simulink model "Simulation5"  (R2020a)
settings: Solver=VariableStepAuto  StartTime=0.0  StopTime=1*60*24  RelTol=1e-3
model workspace (MAT data in the model file):
  hr = 0
  mn = 0
libraries: fl_lib x75, nesl_utility x45, simulink_extras x8
(part 2 of 2)

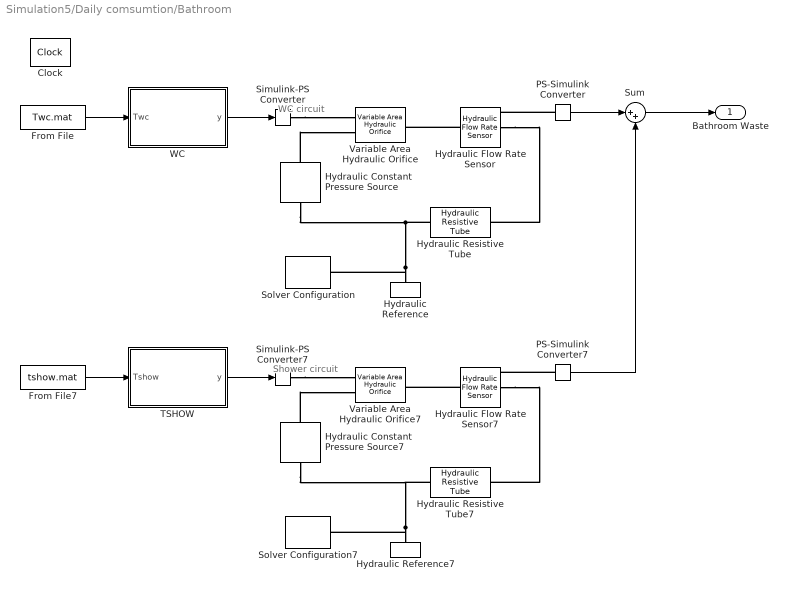
== system Simulation5/Daily comsumtion/Bathroom ==
  note: WC circuit
  note: Shower circuit
  Clock : simulink_extras/Flip Flops/Clock  period=1
  From File : FromFile  FileName=Twc.mat  SampleTime=0
  From File7 : FromFile  FileName=tshow.mat  SampleTime=0
  Hydraulic Constant Pressure Source : fl_lib/Hydraulic/Hydraulic Sources/Hydraulic Constant Pressure Source  commanded_pressure=3 bar
      settings: SourceProductBaseCode=SS  InternalSimscapePortConfiguration="{\"Bottom\":[],\"Left\":[{\"id\":\"P\",\"label\":\"P\",\"type\":\"foundation.hydraulic.hydraulic\"}],\"Right\":[{\"id\":\"T\",\"label\":\"T\",\"type\":\"foundation.hydraulic.hydraulic\"}],\"Top\":[]}"
  Hydraulic Constant Pressure Source7 : fl_lib/Hydraulic/Hydraulic Sources/Hydraulic Constant Pressure Source  commanded_pressure=3 bar
      settings: SourceProductBaseCode=SS  InternalSimscapePortConfiguration="{\"Bottom\":[],\"Left\":[{\"id\":\"P\",\"label\":\"P\",\"type\":\"foundation.hydraulic.hydraulic\"}],\"Right\":[{\"id\":\"T\",\"label\":\"T\",\"type\":\"foundation.hydraulic.hydraulic\"}],\"Top\":[]}"
  Hydraulic Flow Rate Sensor : fl_lib/Hydraulic/Hydraulic Sensors/Hydraulic Flow Rate Sensor
  Hydraulic Flow Rate Sensor7 : fl_lib/Hydraulic/Hydraulic Sensors/Hydraulic Flow Rate Sensor
  Hydraulic Reference : fl_lib/Hydraulic/Hydraulic Elements/Hydraulic Reference
  Hydraulic Reference7 : fl_lib/Hydraulic/Hydraulic Elements/Hydraulic Reference
  Hydraulic Resistive Tube : fl_lib/Hydraulic/Hydraulic Elements/Hydraulic Resistive Tube  cs_type=1  d_in=19 mm  area=1e-4 m^2  D_h=1.12e-2 m  s_factor=0.032  length=17 m  length_ad=1 m  roughness=15e-6 m  Re_lam=2000  Re_turb=4000  q_specify=off  q_priority=None  q=0.001 m^3/s  q_nominal_specify=off  q_nominal_unit=m^3/s  q_nominal_value=1  p_specify=off  p_priority=None  p=0 Pa  p_nominal_specify=off  p_nominal_unit=Pa  p_nominal_value=1
      settings: SourceProductBaseCode=SS  InternalSimscapePortConfiguration="{\"Bottom\":[],\"Left\":[{\"id\":\"A\",\"label\":\"A\",\"type\":\"foundation.hydraulic.hydraulic\"}],\"Right\":[{\"id\":\"B\",\"label\":\"B\",\"type\":\"foundation.hydraulic.hydraulic\"}],\"Top\":[]}"
  Hydraulic Resistive Tube7 : fl_lib/Hydraulic/Hydraulic Elements/Hydraulic Resistive Tube  cs_type=1  d_in=19 mm  area=1e-4 m^2  D_h=1.12e-2 m  s_factor=64  length=17 m  length_ad=1 m  roughness=15e-6 m  Re_lam=2000  Re_turb=4000  q_specify=off  q_priority=None  q=0.001 m^3/s  q_nominal_specify=off  q_nominal_unit=m^3/s  q_nominal_value=1  p_specify=off  p_priority=None  p=0 Pa  p_nominal_specify=off  p_nominal_unit=Pa  p_nominal_value=1
      settings: SourceProductBaseCode=SS  InternalSimscapePortConfiguration="{\"Bottom\":[],\"Left\":[{\"id\":\"A\",\"label\":\"A\",\"type\":\"foundation.hydraulic.hydraulic\"}],\"Right\":[{\"id\":\"B\",\"label\":\"B\",\"type\":\"foundation.hydraulic.hydraulic\"}],\"Top\":[]}"
  PS-Simulink Converter : nesl_utility/PS-Simulink Converter  PhysicalDomain=network_engine_domain  SubClassName=ps_output  LeftPortType=input  RightPortType=output  PseudoPeriodic=off  Frequencies=[]  Unit=1  AffineConversion=off
  PS-Simulink Converter7 : nesl_utility/PS-Simulink Converter  PhysicalDomain=network_engine_domain  SubClassName=ps_output  LeftPortType=input  RightPortType=output  PseudoPeriodic=off  Frequencies=[]  Unit=1  AffineConversion=off
  Simulink-PS Converter : nesl_utility/Simulink-PS Converter  PhysicalDomain=network_engine_domain  SubClassName=ps_input  LeftPortType=input  RightPortType=output  PseudoPeriodic=off  Frequencies=[]  NoiseDistribution=none  NoiseParameters=[]  Unit=1  AffineConversion=off  FilteringAndDerivatives=provide  SimscapeFilterOrder=1  InputFilterTimeConstant=0.001  UdotUserProvided=0
  Simulink-PS Converter7 : nesl_utility/Simulink-PS Converter  PhysicalDomain=network_engine_domain  SubClassName=ps_input  LeftPortType=input  RightPortType=output  PseudoPeriodic=off  Frequencies=[]  NoiseDistribution=none  NoiseParameters=[]  Unit=1  AffineConversion=off  FilteringAndDerivatives=provide  SimscapeFilterOrder=1  InputFilterTimeConstant=0.001  UdotUserProvided=0
  Solver Configuration : nesl_utility/Solver Configuration  PhysicalDomain=network_engine_domain  SubClassName=solver  LeftPortType=input  RightPortType=generic  Tones=[]  Harmonics=[]  SimulateNoise=off  Profile=off  UseLocalSampling=off  EnableSwitchedLinearOptims=on  FrequencyDomain=off  UseCCode=off  RelTol=0.001  AbsTol=1e-06  MinStep=1e-09  ToWorkspace=off  RevertToSquareIcSolve=off  NumHomotopyIterations=100  PhasorMode=off  PhasorModeNumHarmonics=1  DoDC=off  ResidualTolerance=1e-09  UseLocalSolver=off  LocalSolverChoice=NE_BACKWARD_EULER_ADVANCER  LocalSolverSampleTime=0.001  DoFixedCost=off  MaxNonlinIter=3  MaxModeIter=2  LinearAlgebra=auto  EquationFormulation=NE_TIME_EF  DelaysMemoryBudget=1024  AutomaticFiltering=on  FilteringTimeConstant=0.001  PartitionStorageMethod=AS_NEEDED  PartitionMemoryBudget=1024  PartitionMethod=ROBUST
  Solver Configuration7 : nesl_utility/Solver Configuration  PhysicalDomain=network_engine_domain  SubClassName=solver  LeftPortType=input  RightPortType=generic  Tones=[]  Harmonics=[]  SimulateNoise=off  Profile=off  UseLocalSampling=off  EnableSwitchedLinearOptims=on  FrequencyDomain=off  UseCCode=off  RelTol=0.001  AbsTol=1e-06  MinStep=1e-09  ToWorkspace=off  RevertToSquareIcSolve=off  NumHomotopyIterations=100  PhasorMode=off  PhasorModeNumHarmonics=1  DoDC=off  ResidualTolerance=1e-09  UseLocalSolver=off  LocalSolverChoice=NE_BACKWARD_EULER_ADVANCER  LocalSolverSampleTime=0.001  DoFixedCost=off  MaxNonlinIter=3  MaxModeIter=2  LinearAlgebra=auto  EquationFormulation=NE_TIME_EF  DelaysMemoryBudget=1024  AutomaticFiltering=on  FilteringTimeConstant=0.001  PartitionStorageMethod=AS_NEEDED  PartitionMemoryBudget=1024  PartitionMethod=ROBUST
  Sum : Sum  Inputs=|++
  TSHOW : MATLAB Function  TreatAsAtomicUnit=on
  Variable Area Hydraulic Orifice : fl_lib/Hydraulic/Hydraulic Elements/Variable Area Hydraulic Orifice  C_d=0.7  min_area=1e-12 m^2  lam_spec=1  B_lam=0.999  Re_cr=12  q_specify=on  q_priority=None  q=12 lpm  q_nominal_specify=off  q_nominal_unit=m^3/s  q_nominal_value=1  p_specify=off  p_priority=None  p=0 Pa  p_nominal_specify=off  p_nominal_unit=Pa  p_nominal_value=1
      settings: SourceProductBaseCode=SS  InternalSimscapePortConfiguration="{\"Bottom\":[],\"Left\":[{\"id\":\"AR\",\"label\":\"AR\",\"type\":\"input\"},{\"id\":\"A\",\"label\":\"A\",\"type\":\"foundation.hydraulic.hydraulic\"}],\"Right\":[{\"id\":\"B\",\"label\":\"B\",\"type\":\"foundation.hydraulic.hydraulic\"}],\"Top\":[]}"
  Variable Area Hydraulic Orifice7 : fl_lib/Hydraulic/Hydraulic Elements/Variable Area Hydraulic Orifice  C_d=0.7  min_area=1e-12 m^2  lam_spec=1  B_lam=0.999  Re_cr=12  q_specify=on  q_priority=None  q=9 lpm  q_nominal_specify=off  q_nominal_unit=m^3/s  q_nominal_value=1  p_specify=off  p_priority=None  p=0 Pa  p_nominal_specify=off  p_nominal_unit=Pa  p_nominal_value=1
      settings: SourceProductBaseCode=SS  InternalSimscapePortConfiguration="{\"Bottom\":[],\"Left\":[{\"id\":\"AR\",\"label\":\"AR\",\"type\":\"input\"},{\"id\":\"A\",\"label\":\"A\",\"type\":\"foundation.hydraulic.hydraulic\"}],\"Right\":[{\"id\":\"B\",\"label\":\"B\",\"type\":\"foundation.hydraulic.hydraulic\"}],\"Top\":[]}"
  WC : MATLAB Function  TreatAsAtomicUnit=on
  Bathroom Waste : Outport
  wires:
  PS-Simulink Converter/1 -> Sum/1
  TSHOW/1(y) -> Simulink-PS Converter7/1
  From File7/1 -> TSHOW/1(Tshow)
  Sum/1 -> Bathroom Waste/1
  PS-Simulink Converter7/1 -> Sum/2
  WC/1(y) -> Simulink-PS Converter/1
  From File/1 -> WC/1(Twc)
  connections:
  Hydraulic Flow Rate Sensor7/LConn1 -- Variable Area Hydraulic Orifice7/RConn1
  Hydraulic Reference7/LConn1 -- Hydraulic Resistive Tube7/LConn1 -- Hydraulic Constant Pressure Source7/RConn1 -- Solver Configuration7/RConn1
  Hydraulic Flow Rate Sensor/LConn1 -- Variable Area Hydraulic Orifice/RConn1
  Hydraulic Constant Pressure Source7/LConn1 -- Variable Area Hydraulic Orifice7/LConn2
  PS-Simulink Converter7/LConn1 -- Hydraulic Flow Rate Sensor7/RConn1
  Hydraulic Flow Rate Sensor7/RConn2 -- Hydraulic Resistive Tube7/RConn1
  Simulink-PS Converter7/RConn1 -- Variable Area Hydraulic Orifice7/LConn1
  Hydraulic Flow Rate Sensor/RConn2 -- Hydraulic Resistive Tube/RConn1
  PS-Simulink Converter/LConn1 -- Hydraulic Flow Rate Sensor/RConn1
  Hydraulic Resistive Tube/LConn1 -- Hydraulic Constant Pressure Source/RConn1 -- Solver Configuration/RConn1 -- Hydraulic Reference/LConn1
  Hydraulic Constant Pressure Source/LConn1 -- Variable Area Hydraulic Orifice/LConn2
  Simulink-PS Converter/RConn1 -- Variable Area Hydraulic Orifice/LConn1

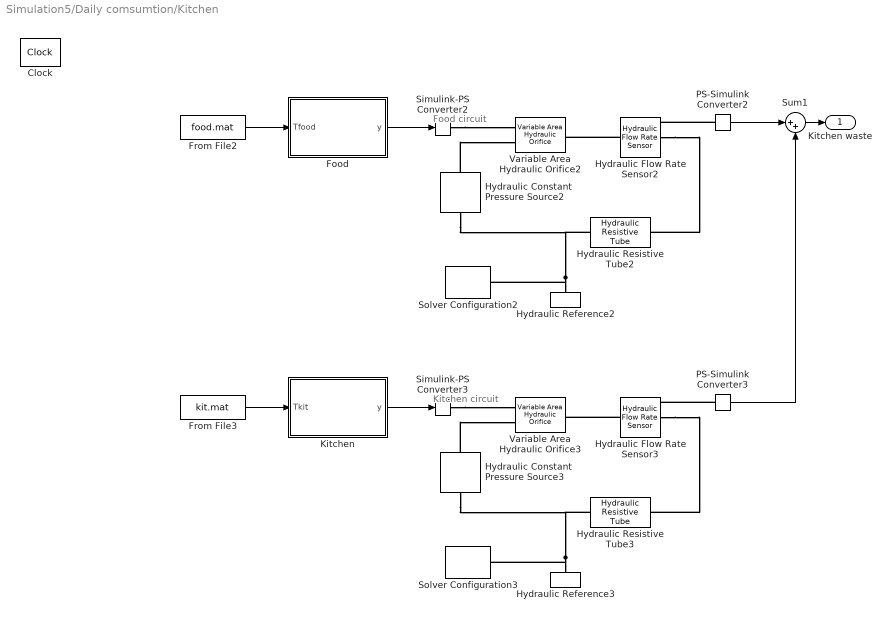
== system Simulation5/Daily comsumtion/Kitchen ==
  note: Food circuit
  note: Kitchen circuit
  Clock : simulink_extras/Flip Flops/Clock  period=1
  Food : MATLAB Function  TreatAsAtomicUnit=on
  From File2 : FromFile  FileName=food.mat  SampleTime=0
  From File3 : FromFile  FileName=kit.mat  SampleTime=0
  Hydraulic Constant Pressure Source2 : fl_lib/Hydraulic/Hydraulic Sources/Hydraulic Constant Pressure Source  commanded_pressure=3 bar
      settings: SourceProductBaseCode=SS  InternalSimscapePortConfiguration="{\"Bottom\":[],\"Left\":[{\"id\":\"P\",\"label\":\"P\",\"type\":\"foundation.hydraulic.hydraulic\"}],\"Right\":[{\"id\":\"T\",\"label\":\"T\",\"type\":\"foundation.hydraulic.hydraulic\"}],\"Top\":[]}"
  Hydraulic Constant Pressure Source3 : fl_lib/Hydraulic/Hydraulic Sources/Hydraulic Constant Pressure Source  commanded_pressure=3 bar
      settings: SourceProductBaseCode=SS  InternalSimscapePortConfiguration="{\"Bottom\":[],\"Left\":[{\"id\":\"P\",\"label\":\"P\",\"type\":\"foundation.hydraulic.hydraulic\"}],\"Right\":[{\"id\":\"T\",\"label\":\"T\",\"type\":\"foundation.hydraulic.hydraulic\"}],\"Top\":[]}"
  Hydraulic Flow Rate Sensor2 : fl_lib/Hydraulic/Hydraulic Sensors/Hydraulic Flow Rate Sensor
  Hydraulic Flow Rate Sensor3 : fl_lib/Hydraulic/Hydraulic Sensors/Hydraulic Flow Rate Sensor
  Hydraulic Reference2 : fl_lib/Hydraulic/Hydraulic Elements/Hydraulic Reference
  Hydraulic Reference3 : fl_lib/Hydraulic/Hydraulic Elements/Hydraulic Reference
  Hydraulic Resistive Tube2 : fl_lib/Hydraulic/Hydraulic Elements/Hydraulic Resistive Tube  cs_type=1  d_in=19 mm  area=1e-4 m^2  D_h=1.12e-2 m  s_factor=0.032  length=8 m  length_ad=1 m  roughness=15e-6 m  Re_lam=2000  Re_turb=4000  q_specify=off  q_priority=None  q=0.001 m^3/s  q_nominal_specify=off  q_nominal_unit=m^3/s  q_nominal_value=1  p_specify=off  p_priority=None  p=0 Pa  p_nominal_specify=off  p_nominal_unit=Pa  p_nominal_value=1
      settings: SourceProductBaseCode=SS  InternalSimscapePortConfiguration="{\"Bottom\":[],\"Left\":[{\"id\":\"A\",\"label\":\"A\",\"type\":\"foundation.hydraulic.hydraulic\"}],\"Right\":[{\"id\":\"B\",\"label\":\"B\",\"type\":\"foundation.hydraulic.hydraulic\"}],\"Top\":[]}"
  Hydraulic Resistive Tube3 : fl_lib/Hydraulic/Hydraulic Elements/Hydraulic Resistive Tube  cs_type=1  d_in=19 mm  area=1e-4 m^2  D_h=1.12e-2 m  s_factor=0.032  length=8 m  length_ad=1 m  roughness=15e-6 m  Re_lam=2000  Re_turb=4000  q_specify=off  q_priority=None  q=0.001 m^3/s  q_nominal_specify=off  q_nominal_unit=m^3/s  q_nominal_value=1  p_specify=off  p_priority=None  p=0 Pa  p_nominal_specify=off  p_nominal_unit=Pa  p_nominal_value=1
      settings: SourceProductBaseCode=SS  InternalSimscapePortConfiguration="{\"Bottom\":[],\"Left\":[{\"id\":\"A\",\"label\":\"A\",\"type\":\"foundation.hydraulic.hydraulic\"}],\"Right\":[{\"id\":\"B\",\"label\":\"B\",\"type\":\"foundation.hydraulic.hydraulic\"}],\"Top\":[]}"
  Kitchen : MATLAB Function  TreatAsAtomicUnit=on
  PS-Simulink Converter2 : nesl_utility/PS-Simulink Converter  PhysicalDomain=network_engine_domain  SubClassName=ps_output  LeftPortType=input  RightPortType=output  PseudoPeriodic=off  Frequencies=[]  Unit=1  AffineConversion=off
  PS-Simulink Converter3 : nesl_utility/PS-Simulink Converter  PhysicalDomain=network_engine_domain  SubClassName=ps_output  LeftPortType=input  RightPortType=output  PseudoPeriodic=off  Frequencies=[]  Unit=1  AffineConversion=off
  Simulink-PS Converter2 : nesl_utility/Simulink-PS Converter  PhysicalDomain=network_engine_domain  SubClassName=ps_input  LeftPortType=input  RightPortType=output  PseudoPeriodic=off  Frequencies=[]  NoiseDistribution=none  NoiseParameters=[]  Unit=1  AffineConversion=off  FilteringAndDerivatives=provide  SimscapeFilterOrder=1  InputFilterTimeConstant=0.001  UdotUserProvided=0
  Simulink-PS Converter3 : nesl_utility/Simulink-PS Converter  PhysicalDomain=network_engine_domain  SubClassName=ps_input  LeftPortType=input  RightPortType=output  PseudoPeriodic=off  Frequencies=[]  NoiseDistribution=none  NoiseParameters=[]  Unit=1  AffineConversion=off  FilteringAndDerivatives=provide  SimscapeFilterOrder=1  InputFilterTimeConstant=0.001  UdotUserProvided=0
  Solver Configuration2 : nesl_utility/Solver Configuration  PhysicalDomain=network_engine_domain  SubClassName=solver  LeftPortType=input  RightPortType=generic  Tones=[]  Harmonics=[]  SimulateNoise=off  Profile=off  UseLocalSampling=off  EnableSwitchedLinearOptims=on  FrequencyDomain=off  UseCCode=off  RelTol=0.001  AbsTol=1e-06  MinStep=1e-09  ToWorkspace=off  RevertToSquareIcSolve=off  NumHomotopyIterations=100  PhasorMode=off  PhasorModeNumHarmonics=1  DoDC=off  ResidualTolerance=1e-09  UseLocalSolver=off  LocalSolverChoice=NE_BACKWARD_EULER_ADVANCER  LocalSolverSampleTime=0.001  DoFixedCost=off  MaxNonlinIter=3  MaxModeIter=2  LinearAlgebra=auto  EquationFormulation=NE_TIME_EF  DelaysMemoryBudget=1024  AutomaticFiltering=on  FilteringTimeConstant=0.001  PartitionStorageMethod=AS_NEEDED  PartitionMemoryBudget=1024  PartitionMethod=ROBUST
  Solver Configuration3 : nesl_utility/Solver Configuration  PhysicalDomain=network_engine_domain  SubClassName=solver  LeftPortType=input  RightPortType=generic  Tones=[]  Harmonics=[]  SimulateNoise=off  Profile=off  UseLocalSampling=off  EnableSwitchedLinearOptims=on  FrequencyDomain=off  UseCCode=off  RelTol=0.001  AbsTol=1e-06  MinStep=1e-09  ToWorkspace=off  RevertToSquareIcSolve=off  NumHomotopyIterations=100  PhasorMode=off  PhasorModeNumHarmonics=1  DoDC=off  ResidualTolerance=1e-09  UseLocalSolver=off  LocalSolverChoice=NE_BACKWARD_EULER_ADVANCER  LocalSolverSampleTime=0.001  DoFixedCost=off  MaxNonlinIter=3  MaxModeIter=2  LinearAlgebra=auto  EquationFormulation=NE_TIME_EF  DelaysMemoryBudget=1024  AutomaticFiltering=on  FilteringTimeConstant=0.001  PartitionStorageMethod=AS_NEEDED  PartitionMemoryBudget=1024  PartitionMethod=ROBUST
  Sum1 : Sum  Inputs=|++
  Variable Area Hydraulic Orifice2 : fl_lib/Hydraulic/Hydraulic Elements/Variable Area Hydraulic Orifice  C_d=0.7  min_area=1e-12 m^2  lam_spec=1  B_lam=0.999  Re_cr=12  q_specify=on  q_priority=None  q=5 lpm  q_nominal_specify=off  q_nominal_unit=m^3/s  q_nominal_value=1  p_specify=off  p_priority=None  p=0 Pa  p_nominal_specify=off  p_nominal_unit=Pa  p_nominal_value=1
      settings: SourceProductBaseCode=SS  InternalSimscapePortConfiguration="{\"Bottom\":[],\"Left\":[{\"id\":\"AR\",\"label\":\"AR\",\"type\":\"input\"},{\"id\":\"A\",\"label\":\"A\",\"type\":\"foundation.hydraulic.hydraulic\"}],\"Right\":[{\"id\":\"B\",\"label\":\"B\",\"type\":\"foundation.hydraulic.hydraulic\"}],\"Top\":[]}"
  Variable Area Hydraulic Orifice3 : fl_lib/Hydraulic/Hydraulic Elements/Variable Area Hydraulic Orifice  C_d=0.7  min_area=1e-12 m^2  lam_spec=1  B_lam=0.999  Re_cr=12  q_specify=on  q_priority=None  q=5 lpm  q_nominal_specify=off  q_nominal_unit=m^3/s  q_nominal_value=1  p_specify=off  p_priority=None  p=0 Pa  p_nominal_specify=off  p_nominal_unit=Pa  p_nominal_value=1
      settings: SourceProductBaseCode=SS  InternalSimscapePortConfiguration="{\"Bottom\":[],\"Left\":[{\"id\":\"AR\",\"label\":\"AR\",\"type\":\"input\"},{\"id\":\"A\",\"label\":\"A\",\"type\":\"foundation.hydraulic.hydraulic\"}],\"Right\":[{\"id\":\"B\",\"label\":\"B\",\"type\":\"foundation.hydraulic.hydraulic\"}],\"Top\":[]}"
  Kitchen waste : Outport
  wires:
  From File3/1 -> Kitchen/1(Tkit)
  Food/1(y) -> Simulink-PS Converter2/1
  PS-Simulink Converter2/1 -> Sum1/1
  From File2/1 -> Food/1(Tfood)
  Kitchen/1(y) -> Simulink-PS Converter3/1
  Sum1/1 -> Kitchen waste/1
  PS-Simulink Converter3/1 -> Sum1/2
  connections:
  Hydraulic Reference3/LConn1 -- Solver Configuration3/RConn1 -- Hydraulic Resistive Tube3/LConn1 -- Hydraulic Constant Pressure Source3/RConn1
  Hydraulic Reference2/LConn1 -- Solver Configuration2/RConn1 -- Hydraulic Resistive Tube2/LConn1 -- Hydraulic Constant Pressure Source2/RConn1
  Hydraulic Constant Pressure Source2/LConn1 -- Variable Area Hydraulic Orifice2/LConn2
  Hydraulic Flow Rate Sensor2/RConn2 -- Hydraulic Resistive Tube2/RConn1
  Hydraulic Flow Rate Sensor3/RConn2 -- Hydraulic Resistive Tube3/RConn1
  PS-Simulink Converter3/LConn1 -- Hydraulic Flow Rate Sensor3/RConn1
  Hydraulic Constant Pressure Source3/LConn1 -- Variable Area Hydraulic Orifice3/LConn2
  Simulink-PS Converter2/RConn1 -- Variable Area Hydraulic Orifice2/LConn1
  PS-Simulink Converter2/LConn1 -- Hydraulic Flow Rate Sensor2/RConn1
  Simulink-PS Converter3/RConn1 -- Variable Area Hydraulic Orifice3/LConn1
  Hydraulic Flow Rate Sensor3/LConn1 -- Variable Area Hydraulic Orifice3/RConn1
  Hydraulic Flow Rate Sensor2/LConn1 -- Variable Area Hydraulic Orifice2/RConn1

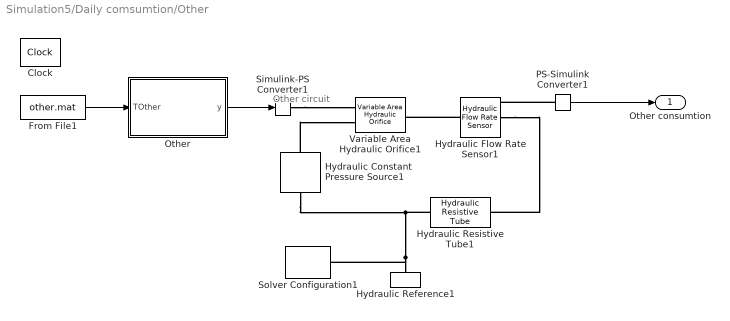
== system Simulation5/Daily comsumtion/Other ==
  note: Other circuit
  Clock : simulink_extras/Flip Flops/Clock  period=1
  From File1 : FromFile  FileName=other.mat  SampleTime=0
  Hydraulic Constant Pressure Source1 : fl_lib/Hydraulic/Hydraulic Sources/Hydraulic Constant Pressure Source  commanded_pressure=3 bar
      settings: SourceProductBaseCode=SS  InternalSimscapePortConfiguration="{\"Bottom\":[],\"Left\":[{\"id\":\"P\",\"label\":\"P\",\"type\":\"foundation.hydraulic.hydraulic\"}],\"Right\":[{\"id\":\"T\",\"label\":\"T\",\"type\":\"foundation.hydraulic.hydraulic\"}],\"Top\":[]}"
  Hydraulic Flow Rate Sensor1 : fl_lib/Hydraulic/Hydraulic Sensors/Hydraulic Flow Rate Sensor
  Hydraulic Reference1 : fl_lib/Hydraulic/Hydraulic Elements/Hydraulic Reference
  Hydraulic Resistive Tube1 : fl_lib/Hydraulic/Hydraulic Elements/Hydraulic Resistive Tube  cs_type=1  d_in=19 mm  area=1e-4 m^2  D_h=1.12e-2 m  s_factor=0.032  length=15 m  length_ad=1 m  roughness=15e-6 m  Re_lam=2000  Re_turb=4000  q_specify=off  q_priority=None  q=0.001 m^3/s  q_nominal_specify=off  q_nominal_unit=m^3/s  q_nominal_value=1  p_specify=off  p_priority=None  p=0 Pa  p_nominal_specify=off  p_nominal_unit=Pa  p_nominal_value=1
      settings: SourceProductBaseCode=SS  InternalSimscapePortConfiguration="{\"Bottom\":[],\"Left\":[{\"id\":\"A\",\"label\":\"A\",\"type\":\"foundation.hydraulic.hydraulic\"}],\"Right\":[{\"id\":\"B\",\"label\":\"B\",\"type\":\"foundation.hydraulic.hydraulic\"}],\"Top\":[]}"
  Other : MATLAB Function  TreatAsAtomicUnit=on
  PS-Simulink Converter1 : nesl_utility/PS-Simulink Converter  PhysicalDomain=network_engine_domain  SubClassName=ps_output  LeftPortType=input  RightPortType=output  PseudoPeriodic=off  Frequencies=[]  Unit=1  AffineConversion=off
  Simulink-PS Converter1 : nesl_utility/Simulink-PS Converter  PhysicalDomain=network_engine_domain  SubClassName=ps_input  LeftPortType=input  RightPortType=output  PseudoPeriodic=off  Frequencies=[]  NoiseDistribution=none  NoiseParameters=[]  Unit=1  AffineConversion=off  FilteringAndDerivatives=provide  SimscapeFilterOrder=1  InputFilterTimeConstant=0.001  UdotUserProvided=0
  Solver Configuration1 : nesl_utility/Solver Configuration  PhysicalDomain=network_engine_domain  SubClassName=solver  LeftPortType=input  RightPortType=generic  Tones=[]  Harmonics=[]  SimulateNoise=off  Profile=off  UseLocalSampling=off  EnableSwitchedLinearOptims=on  FrequencyDomain=off  UseCCode=off  RelTol=0.001  AbsTol=1e-06  MinStep=1e-09  ToWorkspace=off  RevertToSquareIcSolve=off  NumHomotopyIterations=100  PhasorMode=off  PhasorModeNumHarmonics=1  DoDC=off  ResidualTolerance=1e-09  UseLocalSolver=off  LocalSolverChoice=NE_BACKWARD_EULER_ADVANCER  LocalSolverSampleTime=0.001  DoFixedCost=off  MaxNonlinIter=3  MaxModeIter=2  LinearAlgebra=auto  EquationFormulation=NE_TIME_EF  DelaysMemoryBudget=1024  AutomaticFiltering=on  FilteringTimeConstant=0.001  PartitionStorageMethod=AS_NEEDED  PartitionMemoryBudget=1024  PartitionMethod=ROBUST
  Variable Area Hydraulic Orifice1 : fl_lib/Hydraulic/Hydraulic Elements/Variable Area Hydraulic Orifice  C_d=0.7  min_area=1e-12 m^2  lam_spec=1  B_lam=0.999  Re_cr=12  q_specify=on  q_priority=None  q=2.8 lpm  q_nominal_specify=off  q_nominal_unit=m^3/s  q_nominal_value=1  p_specify=off  p_priority=None  p=0 Pa  p_nominal_specify=off  p_nominal_unit=Pa  p_nominal_value=1
      settings: SourceProductBaseCode=SS  InternalSimscapePortConfiguration="{\"Bottom\":[],\"Left\":[{\"id\":\"AR\",\"label\":\"AR\",\"type\":\"input\"},{\"id\":\"A\",\"label\":\"A\",\"type\":\"foundation.hydraulic.hydraulic\"}],\"Right\":[{\"id\":\"B\",\"label\":\"B\",\"type\":\"foundation.hydraulic.hydraulic\"}],\"Top\":[]}"
  Other consumtion : Outport
  wires:
  Other/1(y) -> Simulink-PS Converter1/1
  From File1/1 -> Other/1(TOther)
  PS-Simulink Converter1/1 -> Other consumtion/1
  connections:
  PS-Simulink Converter1/LConn1 -- Hydraulic Flow Rate Sensor1/RConn1
  Hydraulic Flow Rate Sensor1/LConn1 -- Variable Area Hydraulic Orifice1/RConn1
  Hydraulic Constant Pressure Source1/RConn1 -- Hydraulic Resistive Tube1/LConn1 -- Solver Configuration1/RConn1 -- Hydraulic Reference1/LConn1
  Hydraulic Flow Rate Sensor1/RConn2 -- Hydraulic Resistive Tube1/RConn1
  Hydraulic Constant Pressure Source1/LConn1 -- Variable Area Hydraulic Orifice1/LConn2
  Simulink-PS Converter1/RConn1 -- Variable Area Hydraulic Orifice1/LConn1

== matlab function Simulation5/Weekly and fatal Error consumption/Wash ==
  data: Twash input; y output
function y  = Activate(Twash)
    %y=1e-12;
    y=Twash*0.0011/100;
end

== matlab function Simulation5/Weekly and fatal Error consumption/Wash1 ==
  data: Twash input; y output
function y  = Activate(Twash)
    %y=1e-12;
    y=Twash;
end

== matlab function Simulation5/Daily comsumtion/Other/Other ==
  data: TOther input; y output
function y  = Activate(TOther)
    %y=1e-12;
    y=TOther*0.0011;
end

== matlab function Simulation5/Daily comsumtion/Kitchen/Food ==
  data: Tfood input; y output
function y  = Activate(Tfood)
    %y=1e-12;
    y=Tfood*0.0011;
end

== matlab function Simulation5/Daily comsumtion/Kitchen/Kitchen ==
  data: Tkit input; y output
function y  = Activate(Tkit)
    %y=1e-12;
    y=Tkit*0.0011;
end

== matlab function Simulation5/Weekly consumption/Cleani ==
  data: Tcle input; y output
function y  = Activate(Tcle)
    %y=1e-12;
    y=Tcle*0.0011;
end

== matlab function Simulation5/Weekly consumption/Wash ==
  data: Twash input; y output
function y  = Activate(Twash)
    %y=1e-12;
    y=Twash*0.0011;
end

== matlab function Simulation5/Daily Error consumption/Bathroom/TSHOW ==
  data: Tshow input; y output
function y  = Activate(Tshow)
    %y=1e-12;
    y=Tshow*0.0011/100;
end

== matlab function Simulation5/Daily comsumtion/Bathroom/TSHOW ==
  data: Tshow input; y output
function y  = Activate(Tshow)
    %y=1e-12;
    y=Tshow*0.0011;
end

== matlab function Simulation5/Daily Error consumption/Bathroom/WC ==
  data: Twc input; y output
function y  = Activate(Twc)
    %y=1e-12;
    y=Twc*0.0011/100;
end

== matlab function Simulation5/Daily Error consumption/Kitchen/Food ==
  data: Tfood input; y output
function y  = Activate(Tfood)
    %y=1e-12;
    y=Tfood*0.0011/100;
end

== matlab function Simulation5/Daily Error consumption/Kitchen/Kitchen ==
  data: Tkit input; y output
function y  = Activate(Tkit)
    %y=1e-12;
    y=Tkit*0.0011/100;
end

== matlab function Simulation5/Daily Error consumption/Other/Other ==
  data: TOther input; y output
function y  = Activate(TOther)
    %y=1e-12;
    y=TOther*0.0011/100;
end

== matlab function Simulation5/Daily comsumtion/Bathroom/WC ==
  data: Twc input; y output
function y  = Activate(Twc)
    %y=1e-12;
    y=Twc*0.0011;
end

== matlab function Simulation5/Weekly and fatal Error consumption/Cleani ==
  data: Tcle input; y output
function y  = Activate(Tcle)
    %y=1e-12;
    y=Tcle*0.0011/100;
end
